simulink model "EAMP"  (R2023a)
settings: Solver=VariableStepAuto  StartTime=0.0  StopTime=10.0  RelTol=1e-3
settings Model: Creator=paragmraw  LastModifiedBy=paragmraw

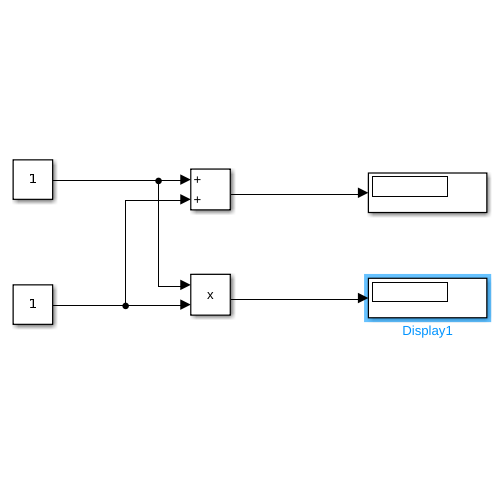
[thumbnail: Simulink's stored preview of the top-level diagram]
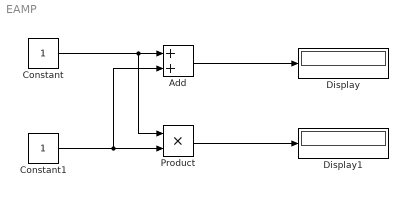
== system EAMP ==
  Add : Sum
  Constant : Constant
  Constant1 : Constant
  Display : Display
  Display1 : Display
  Product : Product
  wires:
  Constant/1 -> Product/1, Add/1
  Constant1/1 -> Product/2, Add/2
  Add/1 -> Display/1
  Product/1 -> Display1/1
